simulink model "CreateFmu_Seperator"  (R2020b)
settings: Solver=FixedStepAuto  StartTime=0.0  StopTime=1  FixedStep=ts  RelTol=1e-3
model workspace (MAT data in the model file):
  ts = 0.01
settings Model: Creator=kaebi  LastModifiedBy=kaebi
settings OptimizationCC: DefaultParameterBehavior=Inlined  LocalBlockOutputs=off
settings RTWCC: GenCodeOnly=on

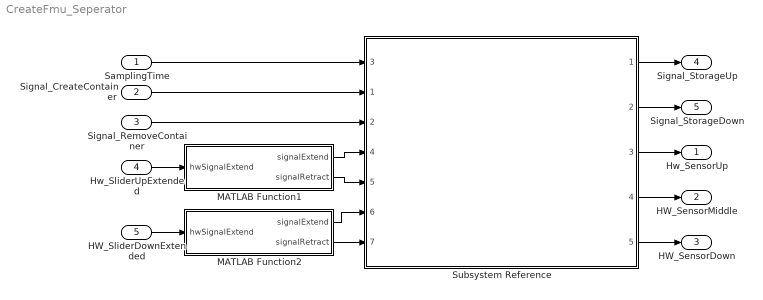
== system CreateFmu_Seperator ==
  SamplingTime : Inport
  Signal_CreateContainer : Inport  Port=2
  Signal_RemoveContainer : Inport  Port=3
  Hw_SliderUpExtended : Inport  Port=4
  HW_SliderDownExtended : Inport  Port=5
  MATLAB Function1 : MATLAB Function  TreatAsAtomicUnit=on
  MATLAB Function2 : MATLAB Function  TreatAsAtomicUnit=on
  Subsystem Reference : Subsystem  ReferencedSubsystem=SubSystemVereinzelung
      settings: PortSchema="{\"entries\":[{\"content\":{\"sides\":[{\"content\":{\"connectorIds\":[\"In3\",\"In1\",\"In2\",\"In4\",\"In5\",\"In6\",\"In7\"]},\"type\":\"ConnectorPlacement.EquallySpacedRectSide\",\"uuid\":\"daf4ed04-6424-45fc-a5e8-18cb4a980d1b\"},{\"content\":{\"connectorIds\":[\"Out1\",\"Out2\",\"Out3\",\"Out4\",\"Out5\"],\"side\":\"RIGHT\"},\"type\":\"ConnectorPlacement.EquallySpacedRectSide\",\"uuid\":\"a47e6a4e-7b46-4a71-a64b-9e4e1f0754a9\"},{\"content\":{\"connectorIds\":[],\"side\":\"TOP\"},\"type\":\"ConnectorPlacement.EquallySpacedRectSide\",\"uuid\":\"b6e6389d-18ca-4ef7-b2f9-2efea5ea42cc\"},{\"content\":{\"connectorIds\":[],\"side\":\"HIDDEN\"},\"type\":\"ConnectorPlacement.EquallySpacedRectSide\",\"uuid\":\"10fc5be0-6c45-4fde-bdc8-b0820f32b2c7\"}]},\"type\":\"ConnectorPlacement.EquallySpacedConnector\",\"uuid\":\"853d100e-9740-4092-b5d4-0ad803ea10a9\"}],\"packageUris\":[\"http://schema.mathworks.com/mf0/Connector/R2020b\"],\"version\":\"1.0\"}"
  Hw_SensorUp : Outport
  HW_SensorMiddle : Outport  Port=2
  HW_SensorDown : Outport  Port=3
  Signal_StorageUp : Outport  Port=4
  Signal_StorageDown : Outport  Port=5
  wires:
  Subsystem Reference/5 -> HW_SensorDown/1
  Subsystem Reference/4 -> HW_SensorMiddle/1
  Subsystem Reference/3 -> Hw_SensorUp/1
  Subsystem Reference/2 -> Signal_StorageDown/1
  Subsystem Reference/1 -> Signal_StorageUp/1
  SamplingTime/1 -> Subsystem Reference/3
  Signal_RemoveContainer/1 -> Subsystem Reference/2
  Signal_CreateContainer/1 -> Subsystem Reference/1
  HW_SliderDownExtended/1 -> MATLAB Function2/1(hwSignalExtend)
  Hw_SliderUpExtended/1 -> MATLAB Function1/1(hwSignalExtend)
  MATLAB Function1/1(signalExtend) -> Subsystem Reference/4
  MATLAB Function1/2(signalRetract) -> Subsystem Reference/5
  MATLAB Function2/1(signalExtend) -> Subsystem Reference/6
  MATLAB Function2/2(signalRetract) -> Subsystem Reference/7

== matlab function CreateFmu_Seperator/MATLAB Function2 ==
  data: hwSignalExtend input; signalExtend output; signalRetract output
function [signalExtend, signalRetract ] = fcn(hwSignalExtend)
    signalExtend = 0;
    signalRetract = 0;

    if (hwSignalExtend >= 1)
        signalExtend = 1;
        signalRetract = 0;
    else
        signalExtend = 0;
        signalRetract = 1;
    end

end

== matlab function CreateFmu_Seperator/MATLAB Function1 ==
  data: hwSignalExtend input; signalExtend output; signalRetract output
function [signalExtend, signalRetract ] = fcn(hwSignalExtend)
    signalExtend = 0;
    signalRetract = 0;

    if (hwSignalExtend >= 1)
        signalExtend = 1;
        signalRetract = 0;
    else
        signalExtend = 0;
        signalRetract = 1;
    end

end
